simulink model "test_NS_NR_SS"  (R2015b)
settings: Solver=VariableStepAuto  StartTime=0.0  StopTime=100  RelTol=1e-3
settings Model: Creator=loicgelle  LastModifiedBy=loicgelle

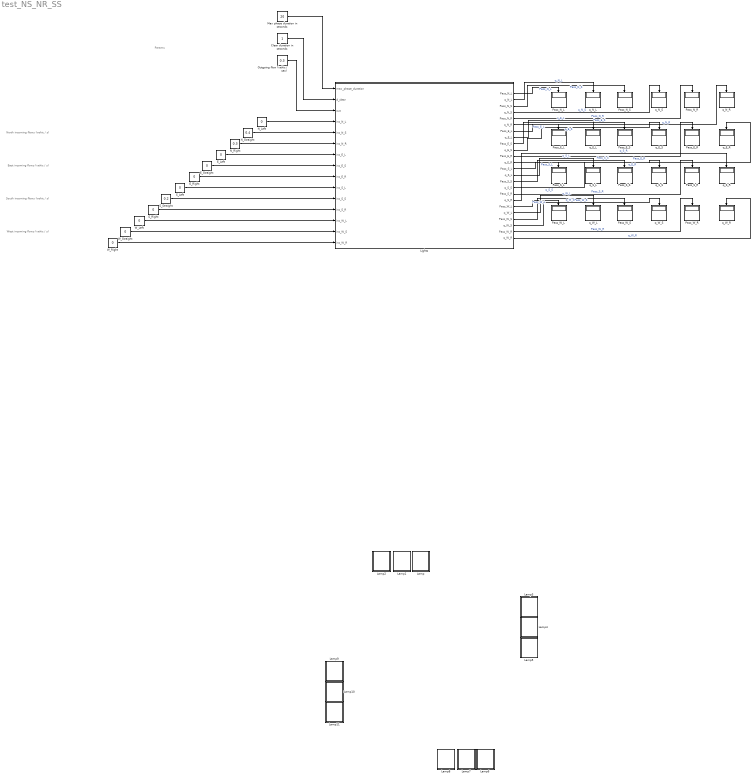
== system test_NS_NR_SS ==
  note: North incoming flows (vehic / s)
  note: East incoming flows (vehic / s)
  note: South incoming flows (vehic / s)
  note: West incoming flows (vehic / s)
  note: Params
  Clear duration in seconds : Constant
  E_Left : Constant  Value=0
  E_Right : Constant  Value=0
  E_Straight : Constant  Value=0
  Lamp : Subsystem  DialogController=hmiCreateDDGDialog  IsWebBlock=on  mask(MWDashboardBlock){webBlockId=bcbba908-b679-4d6f-98d8-b49224a3df23, webBlockType=lamp, ShowInLibBrowser=on, ShowInitialText=on, HMISrcModelName=test_NS_NR_SS}
      mask prompts: webBlockType "WebBlock Type"; HMISrcModelName "Source Model"
      mask Help: helpview([docroot '/mapfiles/simulink.map'], 'hmi_lamp')
      mask Display:
      | if strcmp(get_param(bdroot(gcb),'BlockDiagramType'), 'library')
      |     image([(matlabroot) '/toolbox/simulink/hmi/icons/Lamp.png']);
      | end
  Lamp1 : Subsystem  DialogController=hmiCreateDDGDialog  IsWebBlock=on  mask(MWDashboardBlock){webBlockId=1b688db2-ad5b-4e6b-8226-b397c8e493f7, webBlockType=lamp, ShowInLibBrowser=on, ShowInitialText=on, HMISrcModelName=test_NS_NR_SS}
      mask prompts: webBlockType "WebBlock Type"; HMISrcModelName "Source Model"
      mask Help: helpview([docroot '/mapfiles/simulink.map'], 'hmi_lamp')
      mask Display:
      | if strcmp(get_param(bdroot(gcb),'BlockDiagramType'), 'library')
      |     image([(matlabroot) '/toolbox/simulink/hmi/icons/Lamp.png']);
      | end
  Lamp10 : Subsystem  DialogController=hmiCreateDDGDialog  IsWebBlock=on  mask(MWDashboardBlock){webBlockId=aaceffab-092e-454c-805e-697b255cc4e5, webBlockType=lamp, ShowInLibBrowser=on, ShowInitialText=on, HMISrcModelName=test_NS_NR_SS}
      mask prompts: webBlockType "WebBlock Type"; HMISrcModelName "Source Model"
      mask Help: helpview([docroot '/mapfiles/simulink.map'], 'hmi_lamp')
      mask Display:
      | if strcmp(get_param(bdroot(gcb),'BlockDiagramType'), 'library')
      |     image([(matlabroot) '/toolbox/simulink/hmi/icons/Lamp.png']);
      | end
  Lamp11 : Subsystem  DialogController=hmiCreateDDGDialog  IsWebBlock=on  mask(MWDashboardBlock){webBlockId=6aac982d-ac25-4439-a5bf-feb12f88038f, webBlockType=lamp, ShowInLibBrowser=on, ShowInitialText=on, HMISrcModelName=test_NS_NR_SS}
      mask prompts: webBlockType "WebBlock Type"; HMISrcModelName "Source Model"
      mask Help: helpview([docroot '/mapfiles/simulink.map'], 'hmi_lamp')
      mask Display:
      | if strcmp(get_param(bdroot(gcb),'BlockDiagramType'), 'library')
      |     image([(matlabroot) '/toolbox/simulink/hmi/icons/Lamp.png']);
      | end
  Lamp2 : Subsystem  DialogController=hmiCreateDDGDialog  IsWebBlock=on  mask(MWDashboardBlock){webBlockId=66b2d22a-d359-4ca3-a29d-80af2ca6a62a, webBlockType=lamp, ShowInLibBrowser=on, ShowInitialText=on, HMISrcModelName=test_NS_NR_SS}
      mask prompts: webBlockType "WebBlock Type"; HMISrcModelName "Source Model"
      mask Help: helpview([docroot '/mapfiles/simulink.map'], 'hmi_lamp')
      mask Display:
      | if strcmp(get_param(bdroot(gcb),'BlockDiagramType'), 'library')
      |     image([(matlabroot) '/toolbox/simulink/hmi/icons/Lamp.png']);
      | end
  Lamp3 : Subsystem  DialogController=hmiCreateDDGDialog  IsWebBlock=on  mask(MWDashboardBlock){webBlockId=6276f78b-6ca9-45b4-80e1-6b773a29e60f, webBlockType=lamp, ShowInLibBrowser=on, ShowInitialText=on, HMISrcModelName=test_NS_NR_SS}
      mask prompts: webBlockType "WebBlock Type"; HMISrcModelName "Source Model"
      mask Help: helpview([docroot '/mapfiles/simulink.map'], 'hmi_lamp')
      mask Display:
      | if strcmp(get_param(bdroot(gcb),'BlockDiagramType'), 'library')
      |     image([(matlabroot) '/toolbox/simulink/hmi/icons/Lamp.png']);
      | end
  Lamp4 : Subsystem  DialogController=hmiCreateDDGDialog  IsWebBlock=on  mask(MWDashboardBlock){webBlockId=32819ba0-78ed-40bc-abcc-a791767e98f7, webBlockType=lamp, ShowInLibBrowser=on, ShowInitialText=on, HMISrcModelName=test_NS_NR_SS}
      mask prompts: webBlockType "WebBlock Type"; HMISrcModelName "Source Model"
      mask Help: helpview([docroot '/mapfiles/simulink.map'], 'hmi_lamp')
      mask Display:
      | if strcmp(get_param(bdroot(gcb),'BlockDiagramType'), 'library')
      |     image([(matlabroot) '/toolbox/simulink/hmi/icons/Lamp.png']);
      | end
  Lamp5 : Subsystem  DialogController=hmiCreateDDGDialog  IsWebBlock=on  mask(MWDashboardBlock){webBlockId=42c8e9d6-dd49-4c74-9644-4174f366692c, webBlockType=lamp, ShowInLibBrowser=on, ShowInitialText=on, HMISrcModelName=test_NS_NR_SS}
      mask prompts: webBlockType "WebBlock Type"; HMISrcModelName "Source Model"
      mask Help: helpview([docroot '/mapfiles/simulink.map'], 'hmi_lamp')
      mask Display:
      | if strcmp(get_param(bdroot(gcb),'BlockDiagramType'), 'library')
      |     image([(matlabroot) '/toolbox/simulink/hmi/icons/Lamp.png']);
      | end
  Lamp6 : Subsystem  DialogController=hmiCreateDDGDialog  IsWebBlock=on  mask(MWDashboardBlock){webBlockId=c2314fc7-9623-49b9-8c4b-e96a4599873b, webBlockType=lamp, ShowInLibBrowser=on, ShowInitialText=on, HMISrcModelName=test_NS_NR_SS}
      mask prompts: webBlockType "WebBlock Type"; HMISrcModelName "Source Model"
      mask Help: helpview([docroot '/mapfiles/simulink.map'], 'hmi_lamp')
      mask Display:
      | if strcmp(get_param(bdroot(gcb),'BlockDiagramType'), 'library')
      |     image([(matlabroot) '/toolbox/simulink/hmi/icons/Lamp.png']);
      | end
  Lamp7 : Subsystem  DialogController=hmiCreateDDGDialog  IsWebBlock=on  mask(MWDashboardBlock){webBlockId=8570c1dd-63d7-45c4-ae48-192d725f688d, webBlockType=lamp, ShowInLibBrowser=on, ShowInitialText=on, HMISrcModelName=test_NS_NR_SS}
      mask prompts: webBlockType "WebBlock Type"; HMISrcModelName "Source Model"
      mask Help: helpview([docroot '/mapfiles/simulink.map'], 'hmi_lamp')
      mask Display:
      | if strcmp(get_param(bdroot(gcb),'BlockDiagramType'), 'library')
      |     image([(matlabroot) '/toolbox/simulink/hmi/icons/Lamp.png']);
      | end
  Lamp8 : Subsystem  DialogController=hmiCreateDDGDialog  IsWebBlock=on  mask(MWDashboardBlock){webBlockId=01deec63-d9ed-437d-bf73-454a142b83f1, webBlockType=lamp, ShowInLibBrowser=on, ShowInitialText=on, HMISrcModelName=test_NS_NR_SS}
      mask prompts: webBlockType "WebBlock Type"; HMISrcModelName "Source Model"
      mask Help: helpview([docroot '/mapfiles/simulink.map'], 'hmi_lamp')
      mask Display:
      | if strcmp(get_param(bdroot(gcb),'BlockDiagramType'), 'library')
      |     image([(matlabroot) '/toolbox/simulink/hmi/icons/Lamp.png']);
      | end
  Lamp9 : Subsystem  DialogController=hmiCreateDDGDialog  IsWebBlock=on  mask(MWDashboardBlock){webBlockId=12542d74-6792-45e6-bf4f-ce46703914c2, webBlockType=lamp, ShowInLibBrowser=on, ShowInitialText=on, HMISrcModelName=test_NS_NR_SS}
      mask prompts: webBlockType "WebBlock Type"; HMISrcModelName "Source Model"
      mask Help: helpview([docroot '/mapfiles/simulink.map'], 'hmi_lamp')
      mask Display:
      | if strcmp(get_param(bdroot(gcb),'BlockDiagramType'), 'library')
      |     image([(matlabroot) '/toolbox/simulink/hmi/icons/Lamp.png']);
      | end
  Lights : Stateflow chart  TreatAsAtomicUnit=on  VariantControl=Variant1
  Max phase duration in seconds : Constant  Value=20
  N_Left : Constant  Value=0
  N_Right : Constant  Value=0.3
  N_Straight : Constant  Value=0.4
  Outgoing flow (vehic / sec) : Constant  Value=0.3
  Pass_E_L : Display
  Pass_E_R : Display
  Pass_E_S : Display
  Pass_N_L : Display
  Pass_N_R : Display
  Pass_N_S : Display
  Pass_S_L : Display
  Pass_S_R : Display
  Pass_S_S : Display
  Pass_W_L : Display
  Pass_W_R : Display
  Pass_W_S : Display
  S_Left : Constant  Value=0
  S_Right : Constant  Value=0
  S_Straight : Constant  Value=0.2
  W_Left : Constant  Value=0
  W_Right : Constant  Value=0
  W_Straight : Constant  Value=0
  q_E_L : Display
  q_E_R : Display
  q_E_S : Display
  q_N_L : Display
  q_N_R : Display
  q_N_S : Display
  q_S_L : Display
  q_S_R : Display
  q_S_S : Display
  q_W_L : Display
  q_W_R : Display
  q_W_S : Display
  wires:
  Clear duration in seconds/1 -> Lights/2(d_clear)
  Outgoing flow (vehic / sec)/1 -> Lights/3(out)
  N_Straight/1 -> Lights/5(inc_N_S)
  N_Left/1 -> Lights/4(inc_N_L)
  N_Right/1 -> Lights/6(inc_N_R)
  E_Straight/1 -> Lights/8(inc_E_S)
  E_Right/1 -> Lights/9(inc_E_R)
  E_Left/1 -> Lights/7(inc_E_L)
  S_Straight/1 -> Lights/11(inc_S_S)
  S_Left/1 -> Lights/10(inc_S_L)
  S_Right/1 -> Lights/12(inc_S_R)
  W_Straight/1 -> Lights/14(inc_W_S)
  W_Right/1 -> Lights/15(inc_W_R)
  W_Left/1 -> Lights/13(inc_W_L)
  Lights/1(Pass_N_L) -> Pass_N_L/1  "Pass_N_L"
  Lights/2(q_N_L) -> q_N_L/1  "q_N_L"
  Lights/3(Pass_N_S) -> Pass_N_S/1  "Pass_N_S"
  Lights/4(q_N_S) -> q_N_S/1  "q_N_S"
  Lights/5(Pass_N_R) -> Pass_N_R/1  "Pass_N_R"
  Lights/6(q_N_R) -> q_N_R/1  "q_N_R"
  Lights/7(Pass_E_L) -> Pass_E_L/1  "Pass_E_L"
  Lights/8(q_E_L) -> q_E_L/1  "q_E_L"
  Lights/9(Pass_E_S) -> Pass_E_S/1  "Pass_E_S"
  Lights/10(q_E_S) -> q_E_S/1  "q_E_S"
  Lights/11(Pass_E_R) -> Pass_E_R/1  "Pass_E_R"
  Lights/12(q_E_R) -> q_E_R/1  "q_E_R"
  Lights/13(Pass_S_L) -> Pass_S_L/1  "Pass_S_L"
  Lights/14(q_S_L) -> q_S_L/1  "q_S_L"
  Lights/15(Pass_S_S) -> Pass_S_S/1  "Pass_S_S"
  Lights/16(q_S_S) -> q_S_S/1  "q_S_S"
  Lights/17(Pass_S_R) -> Pass_S_R/1  "Pass_S_R"
  Lights/18(q_S_R) -> q_S_R/1  "q_S_R"
  Lights/19(Pass_W_L) -> Pass_W_L/1  "Pass_W_L"
  Lights/20(q_W_L) -> q_W_L/1  "q_W_L"
  Lights/21(Pass_W_S) -> Pass_W_S/1  "Pass_W_S"
  Lights/22(q_W_S) -> q_W_S/1  "q_W_S"
  Lights/23(Pass_W_R) -> Pass_W_R/1  "Pass_W_R"
  Lights/24(q_W_R) -> q_W_R/1  "q_W_R"
  Max phase duration in seconds/1 -> Lights/1(max_phase_duration)

== system test_NS_NR_SS/Lamp ==

== system test_NS_NR_SS/Lamp1 ==

== system test_NS_NR_SS/Lamp10 ==

== system test_NS_NR_SS/Lamp11 ==

== system test_NS_NR_SS/Lamp2 ==

== system test_NS_NR_SS/Lamp3 ==

== system test_NS_NR_SS/Lamp4 ==

== system test_NS_NR_SS/Lamp5 ==

== system test_NS_NR_SS/Lamp6 ==

== system test_NS_NR_SS/Lamp7 ==

== system test_NS_NR_SS/Lamp8 ==

== system test_NS_NR_SS/Lamp9 ==

== stateflow chart test_NS_NR_SS/Lights ==
  settings: updateMethod=CONTINUOUS
  state QueueHandler_N_L [parallel]
    settings: executionOrder=1
    state Red
      during:
      q_N_L_dot = inc_N_L;
    state Green_Empty
      entry:
      q_N_L = 0;
      during:
      q_N_L_dot = 0;
    state Green
      during:
      q_N_L_dot = inc_N_L - out;
    (default) -> QueueHandler_N_L.Red
    QueueHandler_N_L.Green_Empty -> QueueHandler_N_L.Red [order 2] : [Pass_N_L == 0]
    QueueHandler_N_L.Red -> QueueHandler_N_L.Green : [Pass_N_L == 1]
    QueueHandler_N_L.Green -> QueueHandler_N_L.Red [order 1] : [Pass_N_L == 0]
    QueueHandler_N_L.Green_Empty -> QueueHandler_N_L.Green [order 1] : [out <= inc_N_L]
    QueueHandler_N_L.Green -> QueueHandler_N_L.Green_Empty [order 2] : [q_N_L <= 0 && (out > inc_N_L)]
  state QueueHandler_E_L [parallel]
    settings: executionOrder=5
    state Red
      during:
      q_E_L_dot = inc_E_L;
    state Green_Empty
      entry:
      q_E_L = 0;
      during:
      q_E_L_dot = 0;
    state Green
      during:
      q_E_L_dot = inc_E_L - out;
    (default) -> QueueHandler_E_L.Red
    QueueHandler_E_L.Green_Empty -> QueueHandler_E_L.Red [order 2] : [Pass_E_L == 0]
    QueueHandler_E_L.Red -> QueueHandler_E_L.Green : [Pass_E_L == 1]
    QueueHandler_E_L.Green -> QueueHandler_E_L.Red [order 1] : [Pass_E_L == 0]
    QueueHandler_E_L.Green_Empty -> QueueHandler_E_L.Green [order 1] : [out <= inc_E_L]
    QueueHandler_E_L.Green -> QueueHandler_E_L.Green_Empty [order 2] : [q_E_L <= 0 && (out > inc_E_L)]
  state QueueHandler_S_L [parallel]
    settings: executionOrder=8
    state Red
      during:
      q_S_L_dot = inc_S_L;
    state Green_Empty
      entry:
      q_S_L = 0;
      during:
      q_S_L_dot = 0;
    state Green
      during:
      q_S_L_dot = inc_S_L - out;
    (default) -> QueueHandler_S_L.Red
    QueueHandler_S_L.Green_Empty -> QueueHandler_S_L.Red [order 2] : [Pass_S_L == 0]
    QueueHandler_S_L.Red -> QueueHandler_S_L.Green : [Pass_S_L == 1]
    QueueHandler_S_L.Green -> QueueHandler_S_L.Red [order 1] : [Pass_S_L == 0]
    QueueHandler_S_L.Green_Empty -> QueueHandler_S_L.Green [order 1] : [out <= inc_S_L]
    QueueHandler_S_L.Green -> QueueHandler_S_L.Green_Empty [order 2] : [q_S_L <= 0 && (out > inc_S_L)]
  state QueueHandler_W_L [parallel]
    settings: executionOrder=11
    state Red
      during:
      q_W_L_dot = inc_W_L;
    state Green_Empty
      entry:
      q_W_L = 0;
      during:
      q_W_L_dot = 0;
    state Green
      during:
      q_W_L_dot = inc_W_L - out;
    (default) -> QueueHandler_W_L.Red
    QueueHandler_W_L.Green_Empty -> QueueHandler_W_L.Red [order 2] : [Pass_W_L == 0]
    QueueHandler_W_L.Red -> QueueHandler_W_L.Green : [Pass_W_L == 1]
    QueueHandler_W_L.Green -> QueueHandler_W_L.Red [order 1] : [Pass_W_L == 0]
    QueueHandler_W_L.Green_Empty -> QueueHandler_W_L.Green [order 1] : [out <= inc_W_L]
    QueueHandler_W_L.Green -> QueueHandler_W_L.Green_Empty [order 2] : [q_W_L <= 0 && (out > inc_W_L)]
  state Main_Controller [parallel]
    settings: executionOrder=2
    state Lead_North
      entry:
      t = 0;
      Pass_N_R = 1;
      Pass_N_S = 1;
      Pass_N_L = 1;
      Pass_E_R = 1;
      during:
      t_dot = 1;
      exit:
      Pass_N_R = 0;
      Pass_N_S = 0;
      Pass_N_L = 0;
      Pass_E_R = 0;
      d_N_R = 0;
      d_N_S = 0;
      d_N_L = 0;
      d_E_R = 0;
    state Lead_East
      entry:
      t = 0;
      Pass_E_R = 1;
      Pass_E_S = 1;
      Pass_E_L = 1;
      Pass_S_R = 1;
      during:
      t_dot = 1;
      exit:
      Pass_E_R = 0;
      Pass_E_S = 0;
      Pass_E_L = 0;
      Pass_S_R = 0;
      d_E_R = 0;
      d_E_S = 0;
      d_E_L = 0;
      d_S_R = 0;
    state Lead_South
      entry:
      t = 0;
      Pass_S_R = 1;
      Pass_S_S = 1;
      Pass_S_L = 1;
      Pass_W_R = 1;
      during:
      t_dot = 1;
      exit:
      Pass_S_R = 0;
      Pass_S_S = 0;
      Pass_S_L = 0;
      Pass_W_R = 0;
      d_S_R = 0;
      d_S_S = 0;
      d_S_L = 0;
      d_W_R = 0;
    state Lead_West
      entry:
      t = 0;
      Pass_W_R = 1;
      Pass_W_S = 1;
      Pass_W_L = 1;
      Pass_N_R = 1;
      during:
      t_dot = 1;
      exit:
      Pass_W_R = 0;
      Pass_W_S = 0;
      Pass_W_L = 0;
      Pass_N_R = 0;
      d_W_R = 0;
      d_W_S = 0;
      d_W_L = 0;
      d_N_R = 0;
    state Co_lead_North_South
      entry:
      t = 0;
      Pass_N_R = 1;
      Pass_N_S = 1;
      Pass_S_R = 1;
      Pass_S_S = 1;
      during:
      t_dot = 1;
      exit:
      Pass_N_R = 0;
      Pass_N_S = 0;
      Pass_S_R = 0;
      Pass_S_S = 0;
      d_N_R = 0;
      d_N_S = 0;
      d_S_R = 0;
      d_S_S = 0;
    state Co_lead_East_West
      entry:
      t = 0;
      Pass_E_R = 1;
      Pass_E_S = 1;
      Pass_W_R = 1;
      Pass_W_S = 1;
      during:
      t_dot = 1;
      exit:
      Pass_E_R = 0;
      Pass_E_S = 0;
      Pass_W_R = 0;
      Pass_W_S = 0;
      d_E_R = 0;
      d_E_S = 0;
      d_W_R = 0;
      d_W_S = 0;
    state Semi_lead_North
      entry:
      t = 0;
      Pass_N_R = 1;
      Pass_N_S = 1;
      Pass_E_R = 1;
      Pass_S_R = 1;
      during:
      t_dot = 1;
      exit:
      Pass_N_R = 0;
      Pass_N_S = 0;
      Pass_E_R = 0;
      Pass_S_R = 0;
      d_N_R = 0;
      d_N_S = 0;
      d_E_R = 0;
      d_S_R = 0;
    state Semi_lead_East
      entry:
      t = 0;
      Pass_E_R = 1;
      Pass_E_S = 1;
      Pass_S_R = 1;
      Pass_W_R = 1;
      during:
      t_dot = 1;
      exit:
      Pass_E_R = 0;
      Pass_E_S = 0;
      Pass_S_R = 0;
      Pass_W_R = 0;
      d_E_R = 0;
      d_E_S = 0;
      d_S_R = 0;
      d_W_R = 0;
    state Semi_lead_South
      entry:
      t = 0;
      Pass_S_R = 1;
      Pass_S_S = 1;
      Pass_W_R = 1;
      Pass_N_R = 1;
      during:
      t_dot = 1;
      exit:
      Pass_S_R = 0;
      Pass_S_S = 0;
      Pass_W_R = 0;
      Pass_N_R = 0;
      d_S_R = 0;
      d_S_S = 0;
      d_W_R = 0;
      d_N_R = 0;
    state Semi_lead_West
      entry:
      t = 0;
      Pass_W_R = 1;
      Pass_W_S = 1;
      Pass_N_R = 1;
      Pass_E_R = 1;
      during:
      t_dot = 1;
      exit:
      Pass_W_R = 0;
      Pass_W_S = 0;
      Pass_N_R = 0;
      Pass_E_R = 0;
      d_W_R = 0;
      d_W_S = 0;
      d_N_R = 0;
      d_E_R = 0;
    state Share_Right
      entry:
      t = 0;
      Pass_N_R = 1;
      Pass_E_R = 1;
      Pass_S_R = 1;
      Pass_W_R = 1;
      during:
      t_dot = 1;
      exit:
      Pass_N_R = 0;
      Pass_E_R = 0;
      Pass_S_R = 0;
      Pass_W_R = 0;
      d_N_R = 0;
      d_E_R = 0;
      d_S_R = 0;
      d_W_R = 0;
    state Clear
    Clear -> Share_Right [order 12] : after(d_clear, sec)
        | [ph_code == 11]
    Share_Right -> Clear : [t >= d_phase]
        | {computeNextPhase()}
    Clear -> Semi_lead_North [order 8] : after(d_clear, sec)
        | [ph_code == 7]
    Semi_lead_North -> Clear : [t >= d_phase]
        | {computeNextPhase()}
    Clear -> Lead_North [order 1] : after(d_clear, sec)
        | [ph_code == 1]
    Lead_North -> Clear : [t >= d_phase]
        | {computeNextPhase()}
    Clear -> Lead_East [order 3] : after(d_clear, sec)
        | [ph_code == 2]
    Lead_East -> Clear : [t >= d_phase]
        | {computeNextPhase()}
    Clear -> Lead_West [order 5] : after(d_clear, sec)
        | [ph_code == 4]
    Lead_West -> Clear : [t >= d_phase]
        | {computeNextPhase()}
    Clear -> Co_lead_North_South [order 6] : after(d_clear, sec)
        | [ph_code == 5]
    Co_lead_North_South -> Clear : [t >= d_phase]
        | {computeNextPhase()}
    Clear -> Co_lead_East_West [order 7] : after(d_clear, sec)
        | [ph_code == 6]
    Co_lead_East_West -> Clear : [t >= d_phase]
        | {computeNextPhase()}
    Semi_lead_East -> Clear : [t >= d_phase]
        | {computeNextPhase()}
    Semi_lead_West -> Clear : [t >= d_phase]
        | {computeNextPhase()}
    Clear -> Semi_lead_West [order 11] : after(d_clear, sec)
        | [ph_code == 10]
    Clear -> Semi_lead_South [order 10] : after(d_clear, sec)
        | [ph_code == 9]
    Clear -> Semi_lead_East [order 9] : after(d_clear, sec)
        | [ph_code == 8]
    Semi_lead_South -> Clear : [t >= d_phase]
        | {computeNextPhase()}
    Clear -> Lead_South [order 4] : after(d_clear, sec)
        | [ph_code == 3]
    Lead_South -> Clear : [t >= d_phase]
        | {computeNextPhase()}
    (default) -> Clear : {computeNextPhase()}
    Clear -> Clear [order 2] : after(d_clear, sec)
        | [ph_code == 0]
        | {computeNextPhase()}
  state QueueHandler_N_S [parallel]
    settings: executionOrder=3
    state Red
      during:
      q_N_S_dot = inc_N_S;
    state Green_Empty
      entry:
      q_N_S = 0;
      during:
      q_N_S_dot = 0;
    state Green
      during:
      q_N_S_dot = inc_N_S - out;
    (default) -> QueueHandler_N_S.Red
    QueueHandler_N_S.Green_Empty -> QueueHandler_N_S.Red [order 2] : [Pass_N_S == 0]
    QueueHandler_N_S.Red -> QueueHandler_N_S.Green : [Pass_N_S == 1]
    QueueHandler_N_S.Green -> QueueHandler_N_S.Red [order 1] : [Pass_N_S == 0]
    QueueHandler_N_S.Green_Empty -> QueueHandler_N_S.Green [order 1] : [out <= inc_N_S]
    QueueHandler_N_S.Green -> QueueHandler_N_S.Green_Empty [order 2] : [q_N_S <= 0 && (out > inc_N_S)]
  state QueueHandler_E_S [parallel]
    settings: executionOrder=6
    state Red
      during:
      q_E_S_dot = inc_E_S;
    state Green_Empty
      entry:
      q_E_S = 0;
      during:
      q_E_S_dot = 0;
    state Green
      during:
      q_E_S_dot = inc_E_S - out;
    (default) -> QueueHandler_E_S.Red
    QueueHandler_E_S.Green_Empty -> QueueHandler_E_S.Red [order 2] : [Pass_E_S == 0]
    QueueHandler_E_S.Red -> QueueHandler_E_S.Green : [Pass_E_S == 1]
    QueueHandler_E_S.Green -> QueueHandler_E_S.Red [order 1] : [Pass_E_S == 0]
    QueueHandler_E_S.Green_Empty -> QueueHandler_E_S.Green [order 1] : [out <= inc_E_S]
    QueueHandler_E_S.Green -> QueueHandler_E_S.Green_Empty [order 2] : [q_E_S <= 0 && (out > inc_E_S)]
  state QueueHandler_S_S [parallel]
    settings: executionOrder=9
    state Red
      during:
      q_S_S_dot = inc_S_S;
    state Green_Empty
      entry:
      q_S_S = 0;
      during:
      q_S_S_dot = 0;
    state Green
      during:
      q_S_S_dot = inc_S_S - out;
    (default) -> QueueHandler_S_S.Red
    QueueHandler_S_S.Green_Empty -> QueueHandler_S_S.Red [order 2] : [Pass_S_S == 0]
    QueueHandler_S_S.Red -> QueueHandler_S_S.Green : [Pass_S_S == 1]
    QueueHandler_S_S.Green -> QueueHandler_S_S.Red [order 1] : [Pass_S_S == 0]
    QueueHandler_S_S.Green_Empty -> QueueHandler_S_S.Green [order 1] : [out <= inc_S_S]
    QueueHandler_S_S.Green -> QueueHandler_S_S.Green_Empty [order 2] : [q_S_S <= 0 && (out > inc_S_S)]
  state QueueHandler_W_S [parallel]
    settings: executionOrder=12
    state Red
      during:
      q_W_S_dot = inc_W_S;
    state Green_Empty
      entry:
      q_W_S = 0;
      during:
      q_W_S_dot = 0;
    state Green
      during:
      q_W_S_dot = inc_W_S - out;
    (default) -> QueueHandler_W_S.Red
    QueueHandler_W_S.Green_Empty -> QueueHandler_W_S.Red [order 2] : [Pass_W_S == 0]
    QueueHandler_W_S.Red -> QueueHandler_W_S.Green : [Pass_W_S == 1]
    QueueHandler_W_S.Green -> QueueHandler_W_S.Red [order 1] : [Pass_W_S == 0]
    QueueHandler_W_S.Green -> QueueHandler_W_S.Green_Empty [order 2] : [q_W_S <= 0 && (out > inc_W_S)]
    QueueHandler_W_S.Green_Empty -> QueueHandler_W_S.Green [order 1] : [out <= inc_W_S]
  state QueueHandler_N_R [parallel]
    settings: executionOrder=4
    state Red
      during:
      q_N_R_dot = inc_N_R;
    state Green_Empty
      entry:
      q_N_R = 0;
      during:
      q_N_R_dot = 0;
    state Green
      during:
      q_N_R_dot = inc_N_R - out;
    (default) -> QueueHandler_N_R.Red
    QueueHandler_N_R.Green_Empty -> QueueHandler_N_R.Red [order 2] : [Pass_N_R == 0]
    QueueHandler_N_R.Red -> QueueHandler_N_R.Green : [Pass_N_R == 1]
    QueueHandler_N_R.Green -> QueueHandler_N_R.Red [order 1] : [Pass_N_R == 0]
    QueueHandler_N_R.Green -> QueueHandler_N_R.Green_Empty [order 2] : [q_N_R <= 0 && (out > inc_N_R)]
    QueueHandler_N_R.Green_Empty -> QueueHandler_N_R.Green [order 1] : [out <= inc_N_R]
  state QueueHandler_E_R [parallel]
    settings: executionOrder=7
    state Red
      during:
      q_E_R_dot = inc_E_R;
    state Green_Empty
      entry:
      q_E_R = 0;
      during:
      q_E_R_dot = 0;
    state Green
      during:
      q_E_R_dot = inc_E_R - out;
    (default) -> QueueHandler_E_R.Red
    QueueHandler_E_R.Green_Empty -> QueueHandler_E_R.Red [order 2] : [Pass_E_R == 0]
    QueueHandler_E_R.Red -> QueueHandler_E_R.Green : [Pass_E_R == 1]
    QueueHandler_E_R.Green -> QueueHandler_E_R.Red [order 1] : [Pass_E_R == 0]
    QueueHandler_E_R.Green -> QueueHandler_E_R.Green_Empty [order 2] : [q_E_R <= 0 && (out > inc_E_R)]
    QueueHandler_E_R.Green_Empty -> QueueHandler_E_R.Green [order 1] : [out <= inc_E_R]
  state QueueHandler_S_R [parallel]
    settings: executionOrder=10
    state Red
      during:
      q_S_R_dot = inc_S_R;
    state Green_Empty
      entry:
      q_S_R = 0;
      during:
      q_S_R_dot = 0;
    state Green
      during:
      q_S_R_dot = inc_S_R - out;
    (default) -> QueueHandler_S_R.Red
    QueueHandler_S_R.Green_Empty -> QueueHandler_S_R.Red [order 2] : [Pass_S_R == 0]
    QueueHandler_S_R.Red -> QueueHandler_S_R.Green : [Pass_S_R == 1]
    QueueHandler_S_R.Green -> QueueHandler_S_R.Red [order 1] : [Pass_S_R == 0]
    QueueHandler_S_R.Green -> QueueHandler_S_R.Green_Empty [order 2] : [q_S_R <= 0 && (out > inc_S_R)]
    QueueHandler_S_R.Green_Empty -> QueueHandler_S_R.Green [order 1] : [out <= inc_S_R]
  state QueueHandler_W_R [parallel]
    settings: executionOrder=13
    state Red
      during:
      q_W_R_dot = inc_W_R;
    state Green_Empty
      entry:
      q_W_R = 0;
      during:
      q_W_R_dot = 0;
    state Green
      during:
      q_W_R_dot = inc_W_R - out;
    (default) -> QueueHandler_W_R.Red
    QueueHandler_W_R.Green_Empty -> QueueHandler_W_R.Red [order 2] : [Pass_W_R == 0]
    QueueHandler_W_R.Red -> QueueHandler_W_R.Green : [Pass_W_R == 1]
    QueueHandler_W_R.Green -> QueueHandler_W_R.Red [order 1] : [Pass_W_R == 0]
    QueueHandler_W_R.Green -> QueueHandler_W_R.Green_Empty [order 2] : [q_W_R <= 0 && (out > inc_W_R)]
    QueueHandler_W_R.Green_Empty -> QueueHandler_W_R.Green [order 1] : [out <= inc_W_R]
  data: max_phase_duration input; Pass_N_L output =0; q_N_L output [0..] =0; Pass_N_S output =0; q_N_S output [0..] =0; Pass_N_R output =0; q_N_R output [0..] =0; Pass_E_L output =0; q_E_L output [0..] =0; Pass_E_S output =0; q_E_S output [0..] =0; Pass_E_R output =0; q_E_R output [0..] =0; Pass_S_L output =0; q_S_L output [0..] =0; d_clear input; out input; t local =0; inc_N_L input; inc_N_S input; inc_N_R input; inc_E_L input; inc_E_S input; inc_E_R input; inc_S_L input; inc_S_S input; inc_S_R input; inc_W_L input; inc_W_S input; inc_W_R input; Pass_S_S output =0; q_S_S output [0..] =0; Pass_S_R output =0; q_S_R output [0..] =0; Pass_W_L output =0; q_W_L output [0..] =0; Pass_W_S output =0; q_W_S output [0..] =0; Pass_W_R output =0; q_W_R output [0..] =0; ph_code local =0; d_phase local =0; d_S_S local =1; d_W_S local =1; d_W_L local =1; d_S_L local =1; d_W_R local =1; d_N_R local =1; d_N_S local =1; d_N_L local =1; d_E_R local =1; d_E_S local =1; d_E_L local =1; d_S_R local =1
  data q_N_L settings: updateMethod=SF_CONTINUOUS_TIME_DATA
  data q_N_S settings: updateMethod=SF_CONTINUOUS_TIME_DATA
  data q_N_R settings: updateMethod=SF_CONTINUOUS_TIME_DATA
  data q_E_L settings: updateMethod=SF_CONTINUOUS_TIME_DATA
  data q_E_S settings: updateMethod=SF_CONTINUOUS_TIME_DATA
  data q_E_R settings: updateMethod=SF_CONTINUOUS_TIME_DATA
  data q_S_L settings: updateMethod=SF_CONTINUOUS_TIME_DATA
  data t settings: updateMethod=SF_CONTINUOUS_TIME_DATA
  data q_S_S settings: updateMethod=SF_CONTINUOUS_TIME_DATA
  data q_S_R settings: updateMethod=SF_CONTINUOUS_TIME_DATA
  data q_W_L settings: updateMethod=SF_CONTINUOUS_TIME_DATA
  data q_W_S settings: updateMethod=SF_CONTINUOUS_TIME_DATA
  data q_W_R settings: updateMethod=SF_CONTINUOUS_TIME_DATA
  function computeNextPhase:
    | function computeNextPhase
    | 
    | q_sum_L_N = 3 * q_N_R + 7 * q_N_S + 21 * q_N_L + 3 * q_E_R;
    | q_sum_L_E = 3 * q_E_R + 7 * q_E_S + 21 * q_E_L + 3 * q_S_R;
    | q_sum_L_S = 3 * q_S_R + 7 * q_S_S + 21 * q_S_L + 3 * q_W_R;
    | q_sum_L_W = 3 * q_W_R + 7 * q_W_S + 21 * q_W_L + 3 * q_N_R;
    | q_sum_CL_NS = 3 * q_N_R + 7 * q_N_S + 3 * q_S_R + 7 * q_S_S;
    | q_sum_CL_EW = 3 * q_E_R + 7 * q_E_S + 3 * q_W_R + 7 * q_W_S;
    | q_sum_SL_N = 3 * q_N_R + 7 * q_N_S + 3 * q_S_R + 3 * q_E_R;
    | q_sum_SL_E = 3 * q_E_R + 7 * q_E_S + 3 * q_W_R + 3 * q_S_R;
    | q_sum_SL_S = 3 * q_S_R + 7 * q_S_S + 3 * q_N_R + 3 * q_W_R;
    | q_sum_SL_W = 3 * q_W_R + 7 * q_W_S + 3 * q_E_R + 3 * q_N_R;
    | q_sum_S_R = 3 * q_W_R + 3 * q_E_R + 3 * q_N_R + 3 * q_S_R;
    | 
    | q_max_L_N = max(q_N_R, max(q_N_S, max(q_N_L, q_E_R)));
    | q_max_L_E = max(q_E_R, max(q_E_S, max(q_E_L, q_S_R)));
    | q_max_L_S = max(q_S_R, max(q_S_S, max(q_S_L, q_W_R)));
    | q_max_L_W = max(q_W_R, max(q_W_S, max(q_W_L, q_N_R)));
    | q_max_CL_NS = max(q_N_S, max(q_N_R, max(q_S_S, q_S_R)));
    | q_max_CL_EW = max(q_W_S, max(q_W_R, max(q_E_S, q_E_R)));
    | q_max_SL_N = max(q_N_R, max(q_N_S, max(q_S_R, q_E_R)));
    | q_max_SL_E = max(q_E_R, max(q_E_S, max(q_W_R, q_S_R)));
    | q_max_SL_S = max(q_S_R, max(q_S_S, max(q_N_R, q_W_R)));
    | q_max_SL_W = max(q_W_R, max(q_W_S, max(q_E_R, q_N_R)));
    | q_max_S_R = max(q_N_R, max(q_E_R, max(q_S_R, q_W_R)));
    | 
    | d_sum_L_N = 3 * d_N_R + 7 * d_N_S + 21 * d_N_L + 3 * d_E_R;
    | d_sum_L_E = 3 * d_E_R + 7 * d_E_S + 21 * d_E_L + 3 * d_S_R;
    | d_sum_L_S = 3 * d_S_R + 7 * d_S_S + 21 * d_S_L + 3 * d_W_R;
    | d_sum_L_W = 3 * d_W_R + 7 * d_W_S + 21 * d_W_L + 3 * d_N_R;
    | d_sum_CL_NS = 3 * d_N_R + 7 * d_N_S + 3 * d_S_R + 7 * d_S_S;
    | d_sum_CL_EW = 3 * d_E_R + 7 * d_E_S + 3 * d_W_R + 7 * d_W_S;
    | d_sum_SL_N = 3 * d_N_R + 7 * d_N_S + 3 * d_S_R + 3 * d_E_R;
    | d_sum_SL_E = 3 * d_E_R + 7 * d_E_S + 3 * d_W_R + 3 * d_S_R;
    | d_sum_SL_S = 3 * d_S_R + 7 * d_S_S + 3 * d_N_R + 3 * d_W_R;
    | d_sum_SL_W = 3 * d_W_R + 7 * d_W_S + 3 * d_E_R + 3 * d_N_R;
    | d_sum_S_R = 3 * d_W_R + 3 * d_E_R + 3 * d_N_R + 3 * d_S_R;
    | 
    | q_sum = q_sum_L_N + q_sum_L_E + q_sum_L_S + q_sum_L_W + q_sum_CL_NS + q_sum_CL_EW + q_sum_SL_N + q_sum_SL_E + q_sum_SL_S + q_sum_SL_W + q_sum_S_R;
    | d_sum = d_sum_L_N + d_sum_L_E + d_sum_L_S + d_sum_L_W + d_sum_CL_NS + d_sum_CL_EW + d_sum_SL_N + d_sum_SL_E + d_sum_SL_S + d_sum_SL_W + d_sum_S_R;
    | 
    | coeff_L_N = (d_sum_L_N / d_sum)^2 + (q_sum_L_N / q_sum)^2;
    | coeff_L_E = (d_sum_L_E / d_sum)^2 + (q_sum_L_E / q_sum)^2;
    | coeff_L_S = (d_sum_L_S / d_sum)^2 + (q_sum_L_S / q_sum)^2;
    | coeff_L_W = (d_sum_L_W / d_sum)^2 + (q_sum_L_W / q_sum)^2;
    | coeff_CL_NS = (d_sum_CL_NS / d_sum)^2 + (q_sum_CL_NS / q_sum)^2;
    | coeff_CL_EW = (d_sum_CL_EW / d_sum)^2 + (q_sum_CL_EW / q_sum)^2;
    | coeff_SL_N = (d_sum_SL_N / d_sum)^2 + (q_sum_SL_N / q_sum)^2;
    | coeff_SL_E = (d_sum_SL_E / d_sum)^2 + (q_sum_SL_E / q_sum)^2;
    | coeff_SL_S = (d_sum_SL_S / d_sum)^2 + (q_sum_SL_S / q_sum)^2;
    | coeff_SL_W = (d_sum_SL_W / d_sum)^2 + (q_sum_SL_W / q_sum)^2;
    | coeff_S_R = (d_sum_S_R / d_sum)^2 + (q_sum_S_R / q_sum)^2;
    | 
    | coeff_A = [coeff_L_N, coeff_L_E, coeff_L_S, coeff_L_W, coeff_CL_NS, coeff_CL_EW, coeff_SL_N, coeff_SL_E, coeff_SL_S, coeff_SL_W, coeff_S_R];
    | ix = find(coeff_A == max(coeff_A(:)));
    | 
    | if (q_sum <= 0)
    |     ph_code = 0;
    | elseif any(ix == 1)
    |   ph_code = 1;
    |   d_phase = max(q_max_L_N / out, max_phase_duration);
    | elseif any(ix == 2)
    |   ph_code = 2;
    |   d_phase = max(q_max_L_E / out, max_phase_duration);
    | elseif any(ix == 3)
    |   ph_code = 3;
    |   d_phase = max(q_max_L_S / out, max_phase_duration);
    | elseif any(ix == 4)
    |   ph_code = 4;
    |   d_phase = max(q_max_L_W / out, max_phase_duration);
    | elseif any(ix == 5)
    |   ph_code = 5;
    |   d_phase = max(q_max_CL_NS / out, max_phase_duration);
    | elseif any(ix == 6)
    |   ph_code = 6;
    |   d_phase = max(q_max_CL_EW / out, max_phase_duration);
    | elseif any(ix == 7)
    |   ph_code = 7;
    |   d_phase = max(q_max_SL_N / out, max_phase_duration);
    | elseif any(ix == 8)
    |   ph_coe = 8;
    |   d_phase = max(q_max_SL_E / out, max_phase_duration);
    | elseif any(ix == 9)
    |   ph_code = 9;
    |   d_phase = max(q_max_SL_S / out, max_phase_duration);
    | elseif any(ix == 10)
    |   ph_code = 10;
    |   d_phase = max(q_max_SL_W / out, max_phase_duration);
    | elseif any(ix == 11)
    |   ph_code = 11;
    |   d_phase = max(q_max_S_R / out, max_phase_duration);
    | else
    |   ph_code = 0;
    | end
